simulink model "parallel"  (R2015b)
settings: Solver=FixedStepDiscrete  SolverMode=SingleTasking  StartTime=0.0  StopTime=600e-6  RelTol=1e-3
values from neighbouring files (symbols this model uses):
  b = ['00';'02';'04';'06';'08';'0a';'0c';'0e';'10';'12';'14';'16';'18';'1a';'1c';'1e';'20';'22';'24';'26';'28';'2a';'2c';'2e';'30';'32';'34';'36';'38';'3a';'3c';'3e';'40';'42';'44';'46';'48';'4a';'4c';'4e';'50';'52';'54';'56';'58';'5a';'5c';'5e';'60';'62';'64';'66';'68';'6a';'6c';'6e';'70';'72';'74';'76';'78';'7a';'7c';'7e';'80';'82';'84';'86';'88';'8a';'8c';'8e';'90';'92';'94';'96';'98';'9a';'9c';'9e' ...(+881 chars)    [parallelpipe_tb.m]
  input_sample_rate = 1.0E06    (= 1000000)    [parallelpipe_tb.m]
undefined symbols (not defined in the file or in its folder): a
libraries: shlslibv1 x6037
(part 40 of 40)

== system parallel/AES1 1/Round8/Subsystem8/Subsystem1/Mixcolumn2 ==
  In1 : Inport
  In2 : Inport  Port=2
  In3 : Inport  Port=3
  In4 : Inport  Port=4
  Binary Logic : shlslibv1/Math Functions/Binary Logic  syn_binlog_exp=a^b  synBlockType=primitive  synLatency=0  synBlockId=13
  Binary Logic1 : shlslibv1/Math Functions/Binary Logic  syn_binlog_exp=a^b  synBlockType=primitive  synLatency=0  synBlockId=13
  Binary Logic2 : shlslibv1/Math Functions/Binary Logic  syn_binlog_exp=a^b  synBlockType=primitive  synLatency=0  synBlockId=13
  Display5 : Display
      settings: Format=hex (Stored Integer)
  Port Out : shlslibv1/Ports & Subsystems/Port Out  syn_capture=on  syn_register=on  synBlockType=port  synLatency=1  synBlockId=1
  multiplier2 : shlslibv1/Memories/ROM  syn_rom_vec=multiplier2  syn_rom_auto_wl=on  syn_out_wl=8  syn_out_fl=0  syn_out_dt=unsigned  syn_out_sat=on  syn_out_rnd=on  syn_en_port=off  synBlockType=primitive  synLatency=1  synBlockId=62  syn_dual_port=off
  multiplier3 : shlslibv1/Memories/ROM  syn_rom_vec=multiplier3  syn_rom_auto_wl=on  syn_out_wl=8  syn_out_fl=0  syn_out_dt=unsigned  syn_out_sat=on  syn_out_rnd=on  syn_en_port=off  synBlockType=primitive  synLatency=1  synBlockId=62  syn_dual_port=off
  Out1 : Outport
  wires:
  In1/1 -> Binary Logic/1
  Binary Logic2/1 -> Port Out/1, Out1/1
  In4/1 -> multiplier3/1
  In3/1 -> multiplier2/1
  In2/1 -> Binary Logic/2
  multiplier2/1 -> Binary Logic1/1
  multiplier3/1 -> Binary Logic1/2
  Binary Logic/1 -> Binary Logic2/1
  Binary Logic1/1 -> Binary Logic2/2
  Port Out/1 -> Display5/1

== system parallel/AES1 1/Round8/Subsystem8/Subsystem1/Mixcolumn3 ==
  In1 : Inport
  In2 : Inport  Port=2
  In3 : Inport  Port=3
  In4 : Inport  Port=4
  Binary Logic : shlslibv1/Math Functions/Binary Logic  syn_binlog_exp=a^b  synBlockType=primitive  synLatency=0  synBlockId=13
  Binary Logic1 : shlslibv1/Math Functions/Binary Logic  syn_binlog_exp=a^b  synBlockType=primitive  synLatency=0  synBlockId=13
  Binary Logic2 : shlslibv1/Math Functions/Binary Logic  syn_binlog_exp=a^b  synBlockType=primitive  synLatency=0  synBlockId=13
  Display5 : Display
      settings: Format=hex (Stored Integer)
  Port Out : shlslibv1/Ports & Subsystems/Port Out  syn_capture=on  syn_register=on  synBlockType=port  synLatency=1  synBlockId=1
  multiplier1 : shlslibv1/Memories/ROM  syn_rom_vec=multiplier2  syn_rom_auto_wl=on  syn_out_wl=8  syn_out_fl=0  syn_out_dt=unsigned  syn_out_sat=on  syn_out_rnd=on  syn_en_port=off  synBlockType=primitive  synLatency=1  synBlockId=62  syn_dual_port=off
  multiplier4 : shlslibv1/Memories/ROM  syn_rom_vec=multiplier3  syn_rom_auto_wl=on  syn_out_wl=8  syn_out_fl=0  syn_out_dt=unsigned  syn_out_sat=on  syn_out_rnd=on  syn_en_port=off  synBlockType=primitive  synLatency=1  synBlockId=62  syn_dual_port=off
  Out1 : Outport
  wires:
  In2/1 -> Binary Logic/2
  multiplier1/1 -> Binary Logic1/2
  multiplier4/1 -> Binary Logic/1
  In3/1 -> Binary Logic1/1
  In1/1 -> multiplier4/1
  Binary Logic2/1 -> Port Out/1, Out1/1
  In4/1 -> multiplier1/1
  Port Out/1 -> Display5/1
  Binary Logic/1 -> Binary Logic2/1
  Binary Logic1/1 -> Binary Logic2/2

== system parallel/AES1 1/Round8/Subsystem8/Subsystem2/Mixcolumn ==
  In1 : Inport
  In2 : Inport  Port=2
  In3 : Inport  Port=3
  In4 : Inport  Port=4
  Binary Logic : shlslibv1/Math Functions/Binary Logic  syn_binlog_exp=a^b  synBlockType=primitive  synLatency=0  synBlockId=13
  Binary Logic1 : shlslibv1/Math Functions/Binary Logic  syn_binlog_exp=a^b  synBlockType=primitive  synLatency=0  synBlockId=13
  Binary Logic2 : shlslibv1/Math Functions/Binary Logic  syn_binlog_exp=a^b  synBlockType=primitive  synLatency=0  synBlockId=13
  Display5 : Display
      settings: Format=hex (Stored Integer)
  Port Out : shlslibv1/Ports & Subsystems/Port Out  syn_capture=on  syn_register=on  synBlockType=port  synLatency=1  synBlockId=1
  multiplier2 : shlslibv1/Memories/ROM  syn_rom_vec=multiplier2  syn_rom_auto_wl=on  syn_out_wl=8  syn_out_fl=0  syn_out_dt=unsigned  syn_out_sat=on  syn_out_rnd=on  syn_en_port=off  synBlockType=primitive  synLatency=1  synBlockId=62  syn_dual_port=off
  multiplier3 : shlslibv1/Memories/ROM  syn_rom_vec=multiplier3  syn_rom_auto_wl=on  syn_out_wl=8  syn_out_fl=0  syn_out_dt=unsigned  syn_out_sat=on  syn_out_rnd=on  syn_en_port=off  synBlockType=primitive  synLatency=1  synBlockId=62  syn_dual_port=off
  Out1 : Outport
  wires:
  multiplier3/1 -> Binary Logic/2
  In2/1 -> multiplier3/1
  In4/1 -> Binary Logic1/2
  multiplier2/1 -> Binary Logic/1
  In3/1 -> Binary Logic1/1
  Binary Logic2/1 -> Port Out/1, Out1/1
  In1/1 -> multiplier2/1
  Port Out/1 -> Display5/1
  Binary Logic/1 -> Binary Logic2/1
  Binary Logic1/1 -> Binary Logic2/2

== system parallel/AES1 1/Round8/Subsystem8/Subsystem2/Mixcolumn1 ==
  In1 : Inport
  In2 : Inport  Port=2
  In3 : Inport  Port=3
  In4 : Inport  Port=4
  Binary Logic : shlslibv1/Math Functions/Binary Logic  syn_binlog_exp=a^b  synBlockType=primitive  synLatency=0  synBlockId=13
  Binary Logic1 : shlslibv1/Math Functions/Binary Logic  syn_binlog_exp=a^b  synBlockType=primitive  synLatency=0  synBlockId=13
  Binary Logic2 : shlslibv1/Math Functions/Binary Logic  syn_binlog_exp=a^b  synBlockType=primitive  synLatency=0  synBlockId=13
  Display5 : Display
      settings: Format=hex (Stored Integer)
  Port Out : shlslibv1/Ports & Subsystems/Port Out  syn_capture=on  syn_register=on  synBlockType=port  synLatency=1  synBlockId=1
  multiplier2 : shlslibv1/Memories/ROM  syn_rom_vec=multiplier2  syn_rom_auto_wl=on  syn_out_wl=8  syn_out_fl=0  syn_out_dt=unsigned  syn_out_sat=on  syn_out_rnd=on  syn_en_port=off  synBlockType=primitive  synLatency=1  synBlockId=62  syn_dual_port=off
  multiplier4 : shlslibv1/Memories/ROM  syn_rom_vec=multiplier3  syn_rom_auto_wl=on  syn_out_wl=8  syn_out_fl=0  syn_out_dt=unsigned  syn_out_sat=on  syn_out_rnd=on  syn_en_port=off  synBlockType=primitive  synLatency=1  synBlockId=62  syn_dual_port=off
  Out1 : Outport
  wires:
  multiplier2/1 -> Binary Logic/2
  In2/1 -> multiplier2/1
  In4/1 -> Binary Logic1/2
  In1/1 -> Binary Logic/1
  multiplier4/1 -> Binary Logic1/1
  Binary Logic2/1 -> Port Out/1, Out1/1
  In3/1 -> multiplier4/1
  Port Out/1 -> Display5/1
  Binary Logic/1 -> Binary Logic2/1
  Binary Logic1/1 -> Binary Logic2/2

== system parallel/AES1 1/Round8/Subsystem8/Subsystem2/Mixcolumn2 ==
  In1 : Inport
  In2 : Inport  Port=2
  In3 : Inport  Port=3
  In4 : Inport  Port=4
  Binary Logic : shlslibv1/Math Functions/Binary Logic  syn_binlog_exp=a^b  synBlockType=primitive  synLatency=0  synBlockId=13
  Binary Logic1 : shlslibv1/Math Functions/Binary Logic  syn_binlog_exp=a^b  synBlockType=primitive  synLatency=0  synBlockId=13
  Binary Logic2 : shlslibv1/Math Functions/Binary Logic  syn_binlog_exp=a^b  synBlockType=primitive  synLatency=0  synBlockId=13
  Display5 : Display
      settings: Format=hex (Stored Integer)
  Port Out : shlslibv1/Ports & Subsystems/Port Out  syn_capture=on  syn_register=on  synBlockType=port  synLatency=1  synBlockId=1
  multiplier2 : shlslibv1/Memories/ROM  syn_rom_vec=multiplier2  syn_rom_auto_wl=on  syn_out_wl=8  syn_out_fl=0  syn_out_dt=unsigned  syn_out_sat=on  syn_out_rnd=on  syn_en_port=off  synBlockType=primitive  synLatency=1  synBlockId=62  syn_dual_port=off
  multiplier3 : shlslibv1/Memories/ROM  syn_rom_vec=multiplier3  syn_rom_auto_wl=on  syn_out_wl=8  syn_out_fl=0  syn_out_dt=unsigned  syn_out_sat=on  syn_out_rnd=on  syn_en_port=off  synBlockType=primitive  synLatency=1  synBlockId=62  syn_dual_port=off
  Out1 : Outport
  wires:
  In1/1 -> Binary Logic/1
  Binary Logic2/1 -> Port Out/1, Out1/1
  In4/1 -> multiplier3/1
  In3/1 -> multiplier2/1
  In2/1 -> Binary Logic/2
  multiplier2/1 -> Binary Logic1/1
  multiplier3/1 -> Binary Logic1/2
  Binary Logic/1 -> Binary Logic2/1
  Binary Logic1/1 -> Binary Logic2/2
  Port Out/1 -> Display5/1

== system parallel/AES1 1/Round8/Subsystem8/Subsystem2/Mixcolumn3 ==
  In1 : Inport
  In2 : Inport  Port=2
  In3 : Inport  Port=3
  In4 : Inport  Port=4
  Binary Logic : shlslibv1/Math Functions/Binary Logic  syn_binlog_exp=a^b  synBlockType=primitive  synLatency=0  synBlockId=13
  Binary Logic1 : shlslibv1/Math Functions/Binary Logic  syn_binlog_exp=a^b  synBlockType=primitive  synLatency=0  synBlockId=13
  Binary Logic2 : shlslibv1/Math Functions/Binary Logic  syn_binlog_exp=a^b  synBlockType=primitive  synLatency=0  synBlockId=13
  Display5 : Display
      settings: Format=hex (Stored Integer)
  Port Out : shlslibv1/Ports & Subsystems/Port Out  syn_capture=on  syn_register=on  synBlockType=port  synLatency=1  synBlockId=1
  multiplier1 : shlslibv1/Memories/ROM  syn_rom_vec=multiplier2  syn_rom_auto_wl=on  syn_out_wl=8  syn_out_fl=0  syn_out_dt=unsigned  syn_out_sat=on  syn_out_rnd=on  syn_en_port=off  synBlockType=primitive  synLatency=1  synBlockId=62  syn_dual_port=off
  multiplier4 : shlslibv1/Memories/ROM  syn_rom_vec=multiplier3  syn_rom_auto_wl=on  syn_out_wl=8  syn_out_fl=0  syn_out_dt=unsigned  syn_out_sat=on  syn_out_rnd=on  syn_en_port=off  synBlockType=primitive  synLatency=1  synBlockId=62  syn_dual_port=off
  Out1 : Outport
  wires:
  In2/1 -> Binary Logic/2
  multiplier1/1 -> Binary Logic1/2
  multiplier4/1 -> Binary Logic/1
  In3/1 -> Binary Logic1/1
  In1/1 -> multiplier4/1
  Binary Logic2/1 -> Port Out/1, Out1/1
  In4/1 -> multiplier1/1
  Port Out/1 -> Display5/1
  Binary Logic/1 -> Binary Logic2/1
  Binary Logic1/1 -> Binary Logic2/2

== system parallel/AES1 1/Round8/Subsystem8/Subsystem3/Mixcolumn ==
  In1 : Inport
  In2 : Inport  Port=2
  In3 : Inport  Port=3
  In4 : Inport  Port=4
  Binary Logic : shlslibv1/Math Functions/Binary Logic  syn_binlog_exp=a^b  synBlockType=primitive  synLatency=0  synBlockId=13
  Binary Logic1 : shlslibv1/Math Functions/Binary Logic  syn_binlog_exp=a^b  synBlockType=primitive  synLatency=0  synBlockId=13
  Binary Logic2 : shlslibv1/Math Functions/Binary Logic  syn_binlog_exp=a^b  synBlockType=primitive  synLatency=0  synBlockId=13
  Display5 : Display
      settings: Format=hex (Stored Integer)
  Port Out : shlslibv1/Ports & Subsystems/Port Out  syn_capture=on  syn_register=on  synBlockType=port  synLatency=1  synBlockId=1
  multiplier2 : shlslibv1/Memories/ROM  syn_rom_vec=multiplier2  syn_rom_auto_wl=on  syn_out_wl=8  syn_out_fl=0  syn_out_dt=unsigned  syn_out_sat=on  syn_out_rnd=on  syn_en_port=off  synBlockType=primitive  synLatency=1  synBlockId=62  syn_dual_port=off
  multiplier3 : shlslibv1/Memories/ROM  syn_rom_vec=multiplier3  syn_rom_auto_wl=on  syn_out_wl=8  syn_out_fl=0  syn_out_dt=unsigned  syn_out_sat=on  syn_out_rnd=on  syn_en_port=off  synBlockType=primitive  synLatency=1  synBlockId=62  syn_dual_port=off
  Out1 : Outport
  wires:
  multiplier3/1 -> Binary Logic/2
  In2/1 -> multiplier3/1
  In4/1 -> Binary Logic1/2
  multiplier2/1 -> Binary Logic/1
  In3/1 -> Binary Logic1/1
  Binary Logic2/1 -> Port Out/1, Out1/1
  In1/1 -> multiplier2/1
  Port Out/1 -> Display5/1
  Binary Logic/1 -> Binary Logic2/1
  Binary Logic1/1 -> Binary Logic2/2

== system parallel/AES1 1/Round8/Subsystem8/Subsystem3/Mixcolumn1 ==
  In1 : Inport
  In2 : Inport  Port=2
  In3 : Inport  Port=3
  In4 : Inport  Port=4
  Binary Logic : shlslibv1/Math Functions/Binary Logic  syn_binlog_exp=a^b  synBlockType=primitive  synLatency=0  synBlockId=13
  Binary Logic1 : shlslibv1/Math Functions/Binary Logic  syn_binlog_exp=a^b  synBlockType=primitive  synLatency=0  synBlockId=13
  Binary Logic2 : shlslibv1/Math Functions/Binary Logic  syn_binlog_exp=a^b  synBlockType=primitive  synLatency=0  synBlockId=13
  Display5 : Display
      settings: Format=hex (Stored Integer)
  Port Out : shlslibv1/Ports & Subsystems/Port Out  syn_capture=on  syn_register=on  synBlockType=port  synLatency=1  synBlockId=1
  multiplier2 : shlslibv1/Memories/ROM  syn_rom_vec=multiplier2  syn_rom_auto_wl=on  syn_out_wl=8  syn_out_fl=0  syn_out_dt=unsigned  syn_out_sat=on  syn_out_rnd=on  syn_en_port=off  synBlockType=primitive  synLatency=1  synBlockId=62  syn_dual_port=off
  multiplier4 : shlslibv1/Memories/ROM  syn_rom_vec=multiplier3  syn_rom_auto_wl=on  syn_out_wl=8  syn_out_fl=0  syn_out_dt=unsigned  syn_out_sat=on  syn_out_rnd=on  syn_en_port=off  synBlockType=primitive  synLatency=1  synBlockId=62  syn_dual_port=off
  Out1 : Outport
  wires:
  multiplier2/1 -> Binary Logic/2
  In2/1 -> multiplier2/1
  In4/1 -> Binary Logic1/2
  In1/1 -> Binary Logic/1
  multiplier4/1 -> Binary Logic1/1
  Binary Logic2/1 -> Port Out/1, Out1/1
  In3/1 -> multiplier4/1
  Port Out/1 -> Display5/1
  Binary Logic/1 -> Binary Logic2/1
  Binary Logic1/1 -> Binary Logic2/2

== system parallel/AES1 1/Round8/Subsystem8/Subsystem3/Mixcolumn2 ==
  In1 : Inport
  In2 : Inport  Port=2
  In3 : Inport  Port=3
  In4 : Inport  Port=4
  Binary Logic : shlslibv1/Math Functions/Binary Logic  syn_binlog_exp=a^b  synBlockType=primitive  synLatency=0  synBlockId=13
  Binary Logic1 : shlslibv1/Math Functions/Binary Logic  syn_binlog_exp=a^b  synBlockType=primitive  synLatency=0  synBlockId=13
  Binary Logic2 : shlslibv1/Math Functions/Binary Logic  syn_binlog_exp=a^b  synBlockType=primitive  synLatency=0  synBlockId=13
  Display5 : Display
      settings: Format=hex (Stored Integer)
  Port Out : shlslibv1/Ports & Subsystems/Port Out  syn_capture=on  syn_register=on  synBlockType=port  synLatency=1  synBlockId=1
  multiplier2 : shlslibv1/Memories/ROM  syn_rom_vec=multiplier2  syn_rom_auto_wl=on  syn_out_wl=8  syn_out_fl=0  syn_out_dt=unsigned  syn_out_sat=on  syn_out_rnd=on  syn_en_port=off  synBlockType=primitive  synLatency=1  synBlockId=62  syn_dual_port=off
  multiplier3 : shlslibv1/Memories/ROM  syn_rom_vec=multiplier3  syn_rom_auto_wl=on  syn_out_wl=8  syn_out_fl=0  syn_out_dt=unsigned  syn_out_sat=on  syn_out_rnd=on  syn_en_port=off  synBlockType=primitive  synLatency=1  synBlockId=62  syn_dual_port=off
  Out1 : Outport
  wires:
  In1/1 -> Binary Logic/1
  Binary Logic2/1 -> Port Out/1, Out1/1
  In4/1 -> multiplier3/1
  In3/1 -> multiplier2/1
  In2/1 -> Binary Logic/2
  multiplier2/1 -> Binary Logic1/1
  multiplier3/1 -> Binary Logic1/2
  Binary Logic/1 -> Binary Logic2/1
  Binary Logic1/1 -> Binary Logic2/2
  Port Out/1 -> Display5/1

== system parallel/AES1 1/Round8/Subsystem8/Subsystem3/Mixcolumn3 ==
  In1 : Inport
  In2 : Inport  Port=2
  In3 : Inport  Port=3
  In4 : Inport  Port=4
  Binary Logic : shlslibv1/Math Functions/Binary Logic  syn_binlog_exp=a^b  synBlockType=primitive  synLatency=0  synBlockId=13
  Binary Logic1 : shlslibv1/Math Functions/Binary Logic  syn_binlog_exp=a^b  synBlockType=primitive  synLatency=0  synBlockId=13
  Binary Logic2 : shlslibv1/Math Functions/Binary Logic  syn_binlog_exp=a^b  synBlockType=primitive  synLatency=0  synBlockId=13
  Display5 : Display
      settings: Format=hex (Stored Integer)
  Port Out : shlslibv1/Ports & Subsystems/Port Out  syn_capture=on  syn_register=on  synBlockType=port  synLatency=1  synBlockId=1
  multiplier1 : shlslibv1/Memories/ROM  syn_rom_vec=multiplier2  syn_rom_auto_wl=on  syn_out_wl=8  syn_out_fl=0  syn_out_dt=unsigned  syn_out_sat=on  syn_out_rnd=on  syn_en_port=off  synBlockType=primitive  synLatency=1  synBlockId=62  syn_dual_port=off
  multiplier4 : shlslibv1/Memories/ROM  syn_rom_vec=multiplier3  syn_rom_auto_wl=on  syn_out_wl=8  syn_out_fl=0  syn_out_dt=unsigned  syn_out_sat=on  syn_out_rnd=on  syn_en_port=off  synBlockType=primitive  synLatency=1  synBlockId=62  syn_dual_port=off
  Out1 : Outport
  wires:
  In2/1 -> Binary Logic/2
  multiplier1/1 -> Binary Logic1/2
  multiplier4/1 -> Binary Logic/1
  In3/1 -> Binary Logic1/1
  In1/1 -> multiplier4/1
  Binary Logic2/1 -> Port Out/1, Out1/1
  In4/1 -> multiplier1/1
  Port Out/1 -> Display5/1
  Binary Logic/1 -> Binary Logic2/1
  Binary Logic1/1 -> Binary Logic2/2

== system parallel/AES1 1/Round9/Key1/Keygen1/Subsystem4 ==
  In1 : Inport
  In2 : Inport  Port=2
  In3 : Inport  Port=3
  In4 : Inport  Port=4
  ROM{1..4} (4 alike) : shlslibv1/Memories/ROM  syn_rom_vec=sbox  syn_rom_auto_wl=on  syn_out_wl=8  syn_out_fl=0  syn_out_dt=unsigned  syn_out_sat=on  syn_out_rnd=on  syn_en_port=off  synBlockType=primitive  synLatency=1  synBlockId=62  syn_dual_port=off
  Out1 : Outport
  Out2 : Outport  Port=2
  Out3 : Outport  Port=3
  Out4 : Outport  Port=4
  wires:
  In1/1 -> ROM4/1
  In4/1 -> ROM3/1
  In3/1 -> ROM2/1
  ROM4/1 -> Out1/1
  ROM1/1 -> Out2/1
  ROM2/1 -> Out3/1
  ROM3/1 -> Out4/1
  In2/1 -> ROM1/1

== system parallel/AES1 1/Round9/Subsystem8/Subsystem/Mixcolumn ==
  In1 : Inport
  In2 : Inport  Port=2
  In3 : Inport  Port=3
  In4 : Inport  Port=4
  Binary Logic : shlslibv1/Math Functions/Binary Logic  syn_binlog_exp=a^b  synBlockType=primitive  synLatency=0  synBlockId=13
  Binary Logic1 : shlslibv1/Math Functions/Binary Logic  syn_binlog_exp=a^b  synBlockType=primitive  synLatency=0  synBlockId=13
  Binary Logic2 : shlslibv1/Math Functions/Binary Logic  syn_binlog_exp=a^b  synBlockType=primitive  synLatency=0  synBlockId=13
  Display5 : Display
      settings: Format=hex (Stored Integer)
  Port Out : shlslibv1/Ports & Subsystems/Port Out  syn_capture=on  syn_register=on  synBlockType=port  synLatency=1  synBlockId=1
  multiplier2 : shlslibv1/Memories/ROM  syn_rom_vec=multiplier2  syn_rom_auto_wl=on  syn_out_wl=8  syn_out_fl=0  syn_out_dt=unsigned  syn_out_sat=on  syn_out_rnd=on  syn_en_port=off  synBlockType=primitive  synLatency=1  synBlockId=62  syn_dual_port=off
  multiplier3 : shlslibv1/Memories/ROM  syn_rom_vec=multiplier3  syn_rom_auto_wl=on  syn_out_wl=8  syn_out_fl=0  syn_out_dt=unsigned  syn_out_sat=on  syn_out_rnd=on  syn_en_port=off  synBlockType=primitive  synLatency=1  synBlockId=62  syn_dual_port=off
  Out1 : Outport
  wires:
  multiplier3/1 -> Binary Logic/2
  In2/1 -> multiplier3/1
  In4/1 -> Binary Logic1/2
  multiplier2/1 -> Binary Logic/1
  In3/1 -> Binary Logic1/1
  Binary Logic2/1 -> Port Out/1, Out1/1
  In1/1 -> multiplier2/1
  Port Out/1 -> Display5/1
  Binary Logic/1 -> Binary Logic2/1
  Binary Logic1/1 -> Binary Logic2/2

== system parallel/AES1 1/Round9/Subsystem8/Subsystem/Mixcolumn1 ==
  In1 : Inport
  In2 : Inport  Port=2
  In3 : Inport  Port=3
  In4 : Inport  Port=4
  Binary Logic : shlslibv1/Math Functions/Binary Logic  syn_binlog_exp=a^b  synBlockType=primitive  synLatency=0  synBlockId=13
  Binary Logic1 : shlslibv1/Math Functions/Binary Logic  syn_binlog_exp=a^b  synBlockType=primitive  synLatency=0  synBlockId=13
  Binary Logic2 : shlslibv1/Math Functions/Binary Logic  syn_binlog_exp=a^b  synBlockType=primitive  synLatency=0  synBlockId=13
  Display5 : Display
      settings: Format=hex (Stored Integer)
  Port Out : shlslibv1/Ports & Subsystems/Port Out  syn_capture=on  syn_register=on  synBlockType=port  synLatency=1  synBlockId=1
  multiplier2 : shlslibv1/Memories/ROM  syn_rom_vec=multiplier2  syn_rom_auto_wl=on  syn_out_wl=8  syn_out_fl=0  syn_out_dt=unsigned  syn_out_sat=on  syn_out_rnd=on  syn_en_port=off  synBlockType=primitive  synLatency=1  synBlockId=62  syn_dual_port=off
  multiplier4 : shlslibv1/Memories/ROM  syn_rom_vec=multiplier3  syn_rom_auto_wl=on  syn_out_wl=8  syn_out_fl=0  syn_out_dt=unsigned  syn_out_sat=on  syn_out_rnd=on  syn_en_port=off  synBlockType=primitive  synLatency=1  synBlockId=62  syn_dual_port=off
  Out1 : Outport
  wires:
  multiplier2/1 -> Binary Logic/2
  In2/1 -> multiplier2/1
  In4/1 -> Binary Logic1/2
  In1/1 -> Binary Logic/1
  multiplier4/1 -> Binary Logic1/1
  Binary Logic2/1 -> Port Out/1, Out1/1
  In3/1 -> multiplier4/1
  Port Out/1 -> Display5/1
  Binary Logic/1 -> Binary Logic2/1
  Binary Logic1/1 -> Binary Logic2/2

== system parallel/AES1 1/Round9/Subsystem8/Subsystem/Mixcolumn2 ==
  In1 : Inport
  In2 : Inport  Port=2
  In3 : Inport  Port=3
  In4 : Inport  Port=4
  Binary Logic : shlslibv1/Math Functions/Binary Logic  syn_binlog_exp=a^b  synBlockType=primitive  synLatency=0  synBlockId=13
  Binary Logic1 : shlslibv1/Math Functions/Binary Logic  syn_binlog_exp=a^b  synBlockType=primitive  synLatency=0  synBlockId=13
  Binary Logic2 : shlslibv1/Math Functions/Binary Logic  syn_binlog_exp=a^b  synBlockType=primitive  synLatency=0  synBlockId=13
  Display5 : Display
      settings: Format=hex (Stored Integer)
  Port Out : shlslibv1/Ports & Subsystems/Port Out  syn_capture=on  syn_register=on  synBlockType=port  synLatency=1  synBlockId=1
  multiplier2 : shlslibv1/Memories/ROM  syn_rom_vec=multiplier2  syn_rom_auto_wl=on  syn_out_wl=8  syn_out_fl=0  syn_out_dt=unsigned  syn_out_sat=on  syn_out_rnd=on  syn_en_port=off  synBlockType=primitive  synLatency=1  synBlockId=62  syn_dual_port=off
  multiplier3 : shlslibv1/Memories/ROM  syn_rom_vec=multiplier3  syn_rom_auto_wl=on  syn_out_wl=8  syn_out_fl=0  syn_out_dt=unsigned  syn_out_sat=on  syn_out_rnd=on  syn_en_port=off  synBlockType=primitive  synLatency=1  synBlockId=62  syn_dual_port=off
  Out1 : Outport
  wires:
  In1/1 -> Binary Logic/1
  Binary Logic2/1 -> Port Out/1, Out1/1
  In4/1 -> multiplier3/1
  In3/1 -> multiplier2/1
  In2/1 -> Binary Logic/2
  multiplier2/1 -> Binary Logic1/1
  multiplier3/1 -> Binary Logic1/2
  Binary Logic/1 -> Binary Logic2/1
  Binary Logic1/1 -> Binary Logic2/2
  Port Out/1 -> Display5/1

== system parallel/AES1 1/Round9/Subsystem8/Subsystem/Mixcolumn3 ==
  In1 : Inport
  In2 : Inport  Port=2
  In3 : Inport  Port=3
  In4 : Inport  Port=4
  Binary Logic : shlslibv1/Math Functions/Binary Logic  syn_binlog_exp=a^b  synBlockType=primitive  synLatency=0  synBlockId=13
  Binary Logic1 : shlslibv1/Math Functions/Binary Logic  syn_binlog_exp=a^b  synBlockType=primitive  synLatency=0  synBlockId=13
  Binary Logic2 : shlslibv1/Math Functions/Binary Logic  syn_binlog_exp=a^b  synBlockType=primitive  synLatency=0  synBlockId=13
  Display5 : Display
      settings: Format=hex (Stored Integer)
  Port Out : shlslibv1/Ports & Subsystems/Port Out  syn_capture=on  syn_register=on  synBlockType=port  synLatency=1  synBlockId=1
  multiplier1 : shlslibv1/Memories/ROM  syn_rom_vec=multiplier2  syn_rom_auto_wl=on  syn_out_wl=8  syn_out_fl=0  syn_out_dt=unsigned  syn_out_sat=on  syn_out_rnd=on  syn_en_port=off  synBlockType=primitive  synLatency=1  synBlockId=62  syn_dual_port=off
  multiplier4 : shlslibv1/Memories/ROM  syn_rom_vec=multiplier3  syn_rom_auto_wl=on  syn_out_wl=8  syn_out_fl=0  syn_out_dt=unsigned  syn_out_sat=on  syn_out_rnd=on  syn_en_port=off  synBlockType=primitive  synLatency=1  synBlockId=62  syn_dual_port=off
  Out1 : Outport
  wires:
  In2/1 -> Binary Logic/2
  multiplier1/1 -> Binary Logic1/2
  multiplier4/1 -> Binary Logic/1
  In3/1 -> Binary Logic1/1
  In1/1 -> multiplier4/1
  Binary Logic2/1 -> Port Out/1, Out1/1
  In4/1 -> multiplier1/1
  Port Out/1 -> Display5/1
  Binary Logic/1 -> Binary Logic2/1
  Binary Logic1/1 -> Binary Logic2/2

== system parallel/AES1 1/Round9/Subsystem8/Subsystem1/Mixcolumn ==
  In1 : Inport
  In2 : Inport  Port=2
  In3 : Inport  Port=3
  In4 : Inport  Port=4
  Binary Logic : shlslibv1/Math Functions/Binary Logic  syn_binlog_exp=a^b  synBlockType=primitive  synLatency=0  synBlockId=13
  Binary Logic1 : shlslibv1/Math Functions/Binary Logic  syn_binlog_exp=a^b  synBlockType=primitive  synLatency=0  synBlockId=13
  Binary Logic2 : shlslibv1/Math Functions/Binary Logic  syn_binlog_exp=a^b  synBlockType=primitive  synLatency=0  synBlockId=13
  Display5 : Display
      settings: Format=hex (Stored Integer)
  Port Out : shlslibv1/Ports & Subsystems/Port Out  syn_capture=on  syn_register=on  synBlockType=port  synLatency=1  synBlockId=1
  multiplier2 : shlslibv1/Memories/ROM  syn_rom_vec=multiplier2  syn_rom_auto_wl=on  syn_out_wl=8  syn_out_fl=0  syn_out_dt=unsigned  syn_out_sat=on  syn_out_rnd=on  syn_en_port=off  synBlockType=primitive  synLatency=1  synBlockId=62  syn_dual_port=off
  multiplier3 : shlslibv1/Memories/ROM  syn_rom_vec=multiplier3  syn_rom_auto_wl=on  syn_out_wl=8  syn_out_fl=0  syn_out_dt=unsigned  syn_out_sat=on  syn_out_rnd=on  syn_en_port=off  synBlockType=primitive  synLatency=1  synBlockId=62  syn_dual_port=off
  Out1 : Outport
  wires:
  multiplier3/1 -> Binary Logic/2
  In2/1 -> multiplier3/1
  In4/1 -> Binary Logic1/2
  multiplier2/1 -> Binary Logic/1
  In3/1 -> Binary Logic1/1
  Binary Logic2/1 -> Port Out/1, Out1/1
  In1/1 -> multiplier2/1
  Port Out/1 -> Display5/1
  Binary Logic/1 -> Binary Logic2/1
  Binary Logic1/1 -> Binary Logic2/2

== system parallel/AES1 1/Round9/Subsystem8/Subsystem1/Mixcolumn1 ==
  In1 : Inport
  In2 : Inport  Port=2
  In3 : Inport  Port=3
  In4 : Inport  Port=4
  Binary Logic : shlslibv1/Math Functions/Binary Logic  syn_binlog_exp=a^b  synBlockType=primitive  synLatency=0  synBlockId=13
  Binary Logic1 : shlslibv1/Math Functions/Binary Logic  syn_binlog_exp=a^b  synBlockType=primitive  synLatency=0  synBlockId=13
  Binary Logic2 : shlslibv1/Math Functions/Binary Logic  syn_binlog_exp=a^b  synBlockType=primitive  synLatency=0  synBlockId=13
  Display5 : Display
      settings: Format=hex (Stored Integer)
  Port Out : shlslibv1/Ports & Subsystems/Port Out  syn_capture=on  syn_register=on  synBlockType=port  synLatency=1  synBlockId=1
  multiplier2 : shlslibv1/Memories/ROM  syn_rom_vec=multiplier2  syn_rom_auto_wl=on  syn_out_wl=8  syn_out_fl=0  syn_out_dt=unsigned  syn_out_sat=on  syn_out_rnd=on  syn_en_port=off  synBlockType=primitive  synLatency=1  synBlockId=62  syn_dual_port=off
  multiplier4 : shlslibv1/Memories/ROM  syn_rom_vec=multiplier3  syn_rom_auto_wl=on  syn_out_wl=8  syn_out_fl=0  syn_out_dt=unsigned  syn_out_sat=on  syn_out_rnd=on  syn_en_port=off  synBlockType=primitive  synLatency=1  synBlockId=62  syn_dual_port=off
  Out1 : Outport
  wires:
  multiplier2/1 -> Binary Logic/2
  In2/1 -> multiplier2/1
  In4/1 -> Binary Logic1/2
  In1/1 -> Binary Logic/1
  multiplier4/1 -> Binary Logic1/1
  Binary Logic2/1 -> Port Out/1, Out1/1
  In3/1 -> multiplier4/1
  Port Out/1 -> Display5/1
  Binary Logic/1 -> Binary Logic2/1
  Binary Logic1/1 -> Binary Logic2/2

== system parallel/AES1 1/Round9/Subsystem8/Subsystem1/Mixcolumn2 ==
  In1 : Inport
  In2 : Inport  Port=2
  In3 : Inport  Port=3
  In4 : Inport  Port=4
  Binary Logic : shlslibv1/Math Functions/Binary Logic  syn_binlog_exp=a^b  synBlockType=primitive  synLatency=0  synBlockId=13
  Binary Logic1 : shlslibv1/Math Functions/Binary Logic  syn_binlog_exp=a^b  synBlockType=primitive  synLatency=0  synBlockId=13
  Binary Logic2 : shlslibv1/Math Functions/Binary Logic  syn_binlog_exp=a^b  synBlockType=primitive  synLatency=0  synBlockId=13
  Display5 : Display
      settings: Format=hex (Stored Integer)
  Port Out : shlslibv1/Ports & Subsystems/Port Out  syn_capture=on  syn_register=on  synBlockType=port  synLatency=1  synBlockId=1
  multiplier2 : shlslibv1/Memories/ROM  syn_rom_vec=multiplier2  syn_rom_auto_wl=on  syn_out_wl=8  syn_out_fl=0  syn_out_dt=unsigned  syn_out_sat=on  syn_out_rnd=on  syn_en_port=off  synBlockType=primitive  synLatency=1  synBlockId=62  syn_dual_port=off
  multiplier3 : shlslibv1/Memories/ROM  syn_rom_vec=multiplier3  syn_rom_auto_wl=on  syn_out_wl=8  syn_out_fl=0  syn_out_dt=unsigned  syn_out_sat=on  syn_out_rnd=on  syn_en_port=off  synBlockType=primitive  synLatency=1  synBlockId=62  syn_dual_port=off
  Out1 : Outport
  wires:
  In1/1 -> Binary Logic/1
  Binary Logic2/1 -> Port Out/1, Out1/1
  In4/1 -> multiplier3/1
  In3/1 -> multiplier2/1
  In2/1 -> Binary Logic/2
  multiplier2/1 -> Binary Logic1/1
  multiplier3/1 -> Binary Logic1/2
  Binary Logic/1 -> Binary Logic2/1
  Binary Logic1/1 -> Binary Logic2/2
  Port Out/1 -> Display5/1

== system parallel/AES1 1/Round9/Subsystem8/Subsystem1/Mixcolumn3 ==
  In1 : Inport
  In2 : Inport  Port=2
  In3 : Inport  Port=3
  In4 : Inport  Port=4
  Binary Logic : shlslibv1/Math Functions/Binary Logic  syn_binlog_exp=a^b  synBlockType=primitive  synLatency=0  synBlockId=13
  Binary Logic1 : shlslibv1/Math Functions/Binary Logic  syn_binlog_exp=a^b  synBlockType=primitive  synLatency=0  synBlockId=13
  Binary Logic2 : shlslibv1/Math Functions/Binary Logic  syn_binlog_exp=a^b  synBlockType=primitive  synLatency=0  synBlockId=13
  Display5 : Display
      settings: Format=hex (Stored Integer)
  Port Out : shlslibv1/Ports & Subsystems/Port Out  syn_capture=on  syn_register=on  synBlockType=port  synLatency=1  synBlockId=1
  multiplier1 : shlslibv1/Memories/ROM  syn_rom_vec=multiplier2  syn_rom_auto_wl=on  syn_out_wl=8  syn_out_fl=0  syn_out_dt=unsigned  syn_out_sat=on  syn_out_rnd=on  syn_en_port=off  synBlockType=primitive  synLatency=1  synBlockId=62  syn_dual_port=off
  multiplier4 : shlslibv1/Memories/ROM  syn_rom_vec=multiplier3  syn_rom_auto_wl=on  syn_out_wl=8  syn_out_fl=0  syn_out_dt=unsigned  syn_out_sat=on  syn_out_rnd=on  syn_en_port=off  synBlockType=primitive  synLatency=1  synBlockId=62  syn_dual_port=off
  Out1 : Outport
  wires:
  In2/1 -> Binary Logic/2
  multiplier1/1 -> Binary Logic1/2
  multiplier4/1 -> Binary Logic/1
  In3/1 -> Binary Logic1/1
  In1/1 -> multiplier4/1
  Binary Logic2/1 -> Port Out/1, Out1/1
  In4/1 -> multiplier1/1
  Port Out/1 -> Display5/1
  Binary Logic/1 -> Binary Logic2/1
  Binary Logic1/1 -> Binary Logic2/2

== system parallel/AES1 1/Round9/Subsystem8/Subsystem2/Mixcolumn ==
  In1 : Inport
  In2 : Inport  Port=2
  In3 : Inport  Port=3
  In4 : Inport  Port=4
  Binary Logic : shlslibv1/Math Functions/Binary Logic  syn_binlog_exp=a^b  synBlockType=primitive  synLatency=0  synBlockId=13
  Binary Logic1 : shlslibv1/Math Functions/Binary Logic  syn_binlog_exp=a^b  synBlockType=primitive  synLatency=0  synBlockId=13
  Binary Logic2 : shlslibv1/Math Functions/Binary Logic  syn_binlog_exp=a^b  synBlockType=primitive  synLatency=0  synBlockId=13
  Display5 : Display
      settings: Format=hex (Stored Integer)
  Port Out : shlslibv1/Ports & Subsystems/Port Out  syn_capture=on  syn_register=on  synBlockType=port  synLatency=1  synBlockId=1
  multiplier2 : shlslibv1/Memories/ROM  syn_rom_vec=multiplier2  syn_rom_auto_wl=on  syn_out_wl=8  syn_out_fl=0  syn_out_dt=unsigned  syn_out_sat=on  syn_out_rnd=on  syn_en_port=off  synBlockType=primitive  synLatency=1  synBlockId=62  syn_dual_port=off
  multiplier3 : shlslibv1/Memories/ROM  syn_rom_vec=multiplier3  syn_rom_auto_wl=on  syn_out_wl=8  syn_out_fl=0  syn_out_dt=unsigned  syn_out_sat=on  syn_out_rnd=on  syn_en_port=off  synBlockType=primitive  synLatency=1  synBlockId=62  syn_dual_port=off
  Out1 : Outport
  wires:
  multiplier3/1 -> Binary Logic/2
  In2/1 -> multiplier3/1
  In4/1 -> Binary Logic1/2
  multiplier2/1 -> Binary Logic/1
  In3/1 -> Binary Logic1/1
  Binary Logic2/1 -> Port Out/1, Out1/1
  In1/1 -> multiplier2/1
  Port Out/1 -> Display5/1
  Binary Logic/1 -> Binary Logic2/1
  Binary Logic1/1 -> Binary Logic2/2

== system parallel/AES1 1/Round9/Subsystem8/Subsystem2/Mixcolumn1 ==
  In1 : Inport
  In2 : Inport  Port=2
  In3 : Inport  Port=3
  In4 : Inport  Port=4
  Binary Logic : shlslibv1/Math Functions/Binary Logic  syn_binlog_exp=a^b  synBlockType=primitive  synLatency=0  synBlockId=13
  Binary Logic1 : shlslibv1/Math Functions/Binary Logic  syn_binlog_exp=a^b  synBlockType=primitive  synLatency=0  synBlockId=13
  Binary Logic2 : shlslibv1/Math Functions/Binary Logic  syn_binlog_exp=a^b  synBlockType=primitive  synLatency=0  synBlockId=13
  Display5 : Display
      settings: Format=hex (Stored Integer)
  Port Out : shlslibv1/Ports & Subsystems/Port Out  syn_capture=on  syn_register=on  synBlockType=port  synLatency=1  synBlockId=1
  multiplier2 : shlslibv1/Memories/ROM  syn_rom_vec=multiplier2  syn_rom_auto_wl=on  syn_out_wl=8  syn_out_fl=0  syn_out_dt=unsigned  syn_out_sat=on  syn_out_rnd=on  syn_en_port=off  synBlockType=primitive  synLatency=1  synBlockId=62  syn_dual_port=off
  multiplier4 : shlslibv1/Memories/ROM  syn_rom_vec=multiplier3  syn_rom_auto_wl=on  syn_out_wl=8  syn_out_fl=0  syn_out_dt=unsigned  syn_out_sat=on  syn_out_rnd=on  syn_en_port=off  synBlockType=primitive  synLatency=1  synBlockId=62  syn_dual_port=off
  Out1 : Outport
  wires:
  multiplier2/1 -> Binary Logic/2
  In2/1 -> multiplier2/1
  In4/1 -> Binary Logic1/2
  In1/1 -> Binary Logic/1
  multiplier4/1 -> Binary Logic1/1
  Binary Logic2/1 -> Port Out/1, Out1/1
  In3/1 -> multiplier4/1
  Port Out/1 -> Display5/1
  Binary Logic/1 -> Binary Logic2/1
  Binary Logic1/1 -> Binary Logic2/2

== system parallel/AES1 1/Round9/Subsystem8/Subsystem2/Mixcolumn2 ==
  In1 : Inport
  In2 : Inport  Port=2
  In3 : Inport  Port=3
  In4 : Inport  Port=4
  Binary Logic : shlslibv1/Math Functions/Binary Logic  syn_binlog_exp=a^b  synBlockType=primitive  synLatency=0  synBlockId=13
  Binary Logic1 : shlslibv1/Math Functions/Binary Logic  syn_binlog_exp=a^b  synBlockType=primitive  synLatency=0  synBlockId=13
  Binary Logic2 : shlslibv1/Math Functions/Binary Logic  syn_binlog_exp=a^b  synBlockType=primitive  synLatency=0  synBlockId=13
  Display5 : Display
      settings: Format=hex (Stored Integer)
  Port Out : shlslibv1/Ports & Subsystems/Port Out  syn_capture=on  syn_register=on  synBlockType=port  synLatency=1  synBlockId=1
  multiplier2 : shlslibv1/Memories/ROM  syn_rom_vec=multiplier2  syn_rom_auto_wl=on  syn_out_wl=8  syn_out_fl=0  syn_out_dt=unsigned  syn_out_sat=on  syn_out_rnd=on  syn_en_port=off  synBlockType=primitive  synLatency=1  synBlockId=62  syn_dual_port=off
  multiplier3 : shlslibv1/Memories/ROM  syn_rom_vec=multiplier3  syn_rom_auto_wl=on  syn_out_wl=8  syn_out_fl=0  syn_out_dt=unsigned  syn_out_sat=on  syn_out_rnd=on  syn_en_port=off  synBlockType=primitive  synLatency=1  synBlockId=62  syn_dual_port=off
  Out1 : Outport
  wires:
  In1/1 -> Binary Logic/1
  Binary Logic2/1 -> Port Out/1, Out1/1
  In4/1 -> multiplier3/1
  In3/1 -> multiplier2/1
  In2/1 -> Binary Logic/2
  multiplier2/1 -> Binary Logic1/1
  multiplier3/1 -> Binary Logic1/2
  Binary Logic/1 -> Binary Logic2/1
  Binary Logic1/1 -> Binary Logic2/2
  Port Out/1 -> Display5/1

== system parallel/AES1 1/Round9/Subsystem8/Subsystem2/Mixcolumn3 ==
  In1 : Inport
  In2 : Inport  Port=2
  In3 : Inport  Port=3
  In4 : Inport  Port=4
  Binary Logic : shlslibv1/Math Functions/Binary Logic  syn_binlog_exp=a^b  synBlockType=primitive  synLatency=0  synBlockId=13
  Binary Logic1 : shlslibv1/Math Functions/Binary Logic  syn_binlog_exp=a^b  synBlockType=primitive  synLatency=0  synBlockId=13
  Binary Logic2 : shlslibv1/Math Functions/Binary Logic  syn_binlog_exp=a^b  synBlockType=primitive  synLatency=0  synBlockId=13
  Display5 : Display
      settings: Format=hex (Stored Integer)
  Port Out : shlslibv1/Ports & Subsystems/Port Out  syn_capture=on  syn_register=on  synBlockType=port  synLatency=1  synBlockId=1
  multiplier1 : shlslibv1/Memories/ROM  syn_rom_vec=multiplier2  syn_rom_auto_wl=on  syn_out_wl=8  syn_out_fl=0  syn_out_dt=unsigned  syn_out_sat=on  syn_out_rnd=on  syn_en_port=off  synBlockType=primitive  synLatency=1  synBlockId=62  syn_dual_port=off
  multiplier4 : shlslibv1/Memories/ROM  syn_rom_vec=multiplier3  syn_rom_auto_wl=on  syn_out_wl=8  syn_out_fl=0  syn_out_dt=unsigned  syn_out_sat=on  syn_out_rnd=on  syn_en_port=off  synBlockType=primitive  synLatency=1  synBlockId=62  syn_dual_port=off
  Out1 : Outport
  wires:
  In2/1 -> Binary Logic/2
  multiplier1/1 -> Binary Logic1/2
  multiplier4/1 -> Binary Logic/1
  In3/1 -> Binary Logic1/1
  In1/1 -> multiplier4/1
  Binary Logic2/1 -> Port Out/1, Out1/1
  In4/1 -> multiplier1/1
  Port Out/1 -> Display5/1
  Binary Logic/1 -> Binary Logic2/1
  Binary Logic1/1 -> Binary Logic2/2

== system parallel/AES1 1/Round9/Subsystem8/Subsystem3/Mixcolumn ==
  In1 : Inport
  In2 : Inport  Port=2
  In3 : Inport  Port=3
  In4 : Inport  Port=4
  Binary Logic : shlslibv1/Math Functions/Binary Logic  syn_binlog_exp=a^b  synBlockType=primitive  synLatency=0  synBlockId=13
  Binary Logic1 : shlslibv1/Math Functions/Binary Logic  syn_binlog_exp=a^b  synBlockType=primitive  synLatency=0  synBlockId=13
  Binary Logic2 : shlslibv1/Math Functions/Binary Logic  syn_binlog_exp=a^b  synBlockType=primitive  synLatency=0  synBlockId=13
  Display5 : Display
      settings: Format=hex (Stored Integer)
  Port Out : shlslibv1/Ports & Subsystems/Port Out  syn_capture=on  syn_register=on  synBlockType=port  synLatency=1  synBlockId=1
  multiplier2 : shlslibv1/Memories/ROM  syn_rom_vec=multiplier2  syn_rom_auto_wl=on  syn_out_wl=8  syn_out_fl=0  syn_out_dt=unsigned  syn_out_sat=on  syn_out_rnd=on  syn_en_port=off  synBlockType=primitive  synLatency=1  synBlockId=62  syn_dual_port=off
  multiplier3 : shlslibv1/Memories/ROM  syn_rom_vec=multiplier3  syn_rom_auto_wl=on  syn_out_wl=8  syn_out_fl=0  syn_out_dt=unsigned  syn_out_sat=on  syn_out_rnd=on  syn_en_port=off  synBlockType=primitive  synLatency=1  synBlockId=62  syn_dual_port=off
  Out1 : Outport
  wires:
  multiplier3/1 -> Binary Logic/2
  In2/1 -> multiplier3/1
  In4/1 -> Binary Logic1/2
  multiplier2/1 -> Binary Logic/1
  In3/1 -> Binary Logic1/1
  Binary Logic2/1 -> Port Out/1, Out1/1
  In1/1 -> multiplier2/1
  Port Out/1 -> Display5/1
  Binary Logic/1 -> Binary Logic2/1
  Binary Logic1/1 -> Binary Logic2/2

== system parallel/AES1 1/Round9/Subsystem8/Subsystem3/Mixcolumn1 ==
  In1 : Inport
  In2 : Inport  Port=2
  In3 : Inport  Port=3
  In4 : Inport  Port=4
  Binary Logic : shlslibv1/Math Functions/Binary Logic  syn_binlog_exp=a^b  synBlockType=primitive  synLatency=0  synBlockId=13
  Binary Logic1 : shlslibv1/Math Functions/Binary Logic  syn_binlog_exp=a^b  synBlockType=primitive  synLatency=0  synBlockId=13
  Binary Logic2 : shlslibv1/Math Functions/Binary Logic  syn_binlog_exp=a^b  synBlockType=primitive  synLatency=0  synBlockId=13
  Display5 : Display
      settings: Format=hex (Stored Integer)
  Port Out : shlslibv1/Ports & Subsystems/Port Out  syn_capture=on  syn_register=on  synBlockType=port  synLatency=1  synBlockId=1
  multiplier2 : shlslibv1/Memories/ROM  syn_rom_vec=multiplier2  syn_rom_auto_wl=on  syn_out_wl=8  syn_out_fl=0  syn_out_dt=unsigned  syn_out_sat=on  syn_out_rnd=on  syn_en_port=off  synBlockType=primitive  synLatency=1  synBlockId=62  syn_dual_port=off
  multiplier4 : shlslibv1/Memories/ROM  syn_rom_vec=multiplier3  syn_rom_auto_wl=on  syn_out_wl=8  syn_out_fl=0  syn_out_dt=unsigned  syn_out_sat=on  syn_out_rnd=on  syn_en_port=off  synBlockType=primitive  synLatency=1  synBlockId=62  syn_dual_port=off
  Out1 : Outport
  wires:
  multiplier2/1 -> Binary Logic/2
  In2/1 -> multiplier2/1
  In4/1 -> Binary Logic1/2
  In1/1 -> Binary Logic/1
  multiplier4/1 -> Binary Logic1/1
  Binary Logic2/1 -> Port Out/1, Out1/1
  In3/1 -> multiplier4/1
  Port Out/1 -> Display5/1
  Binary Logic/1 -> Binary Logic2/1
  Binary Logic1/1 -> Binary Logic2/2

== system parallel/AES1 1/Round9/Subsystem8/Subsystem3/Mixcolumn2 ==
  In1 : Inport
  In2 : Inport  Port=2
  In3 : Inport  Port=3
  In4 : Inport  Port=4
  Binary Logic : shlslibv1/Math Functions/Binary Logic  syn_binlog_exp=a^b  synBlockType=primitive  synLatency=0  synBlockId=13
  Binary Logic1 : shlslibv1/Math Functions/Binary Logic  syn_binlog_exp=a^b  synBlockType=primitive  synLatency=0  synBlockId=13
  Binary Logic2 : shlslibv1/Math Functions/Binary Logic  syn_binlog_exp=a^b  synBlockType=primitive  synLatency=0  synBlockId=13
  Display5 : Display
      settings: Format=hex (Stored Integer)
  Port Out : shlslibv1/Ports & Subsystems/Port Out  syn_capture=on  syn_register=on  synBlockType=port  synLatency=1  synBlockId=1
  multiplier2 : shlslibv1/Memories/ROM  syn_rom_vec=multiplier2  syn_rom_auto_wl=on  syn_out_wl=8  syn_out_fl=0  syn_out_dt=unsigned  syn_out_sat=on  syn_out_rnd=on  syn_en_port=off  synBlockType=primitive  synLatency=1  synBlockId=62  syn_dual_port=off
  multiplier3 : shlslibv1/Memories/ROM  syn_rom_vec=multiplier3  syn_rom_auto_wl=on  syn_out_wl=8  syn_out_fl=0  syn_out_dt=unsigned  syn_out_sat=on  syn_out_rnd=on  syn_en_port=off  synBlockType=primitive  synLatency=1  synBlockId=62  syn_dual_port=off
  Out1 : Outport
  wires:
  In1/1 -> Binary Logic/1
  Binary Logic2/1 -> Port Out/1, Out1/1
  In4/1 -> multiplier3/1
  In3/1 -> multiplier2/1
  In2/1 -> Binary Logic/2
  multiplier2/1 -> Binary Logic1/1
  multiplier3/1 -> Binary Logic1/2
  Binary Logic/1 -> Binary Logic2/1
  Binary Logic1/1 -> Binary Logic2/2
  Port Out/1 -> Display5/1

== system parallel/AES1 1/Round9/Subsystem8/Subsystem3/Mixcolumn3 ==
  In1 : Inport
  In2 : Inport  Port=2
  In3 : Inport  Port=3
  In4 : Inport  Port=4
  Binary Logic : shlslibv1/Math Functions/Binary Logic  syn_binlog_exp=a^b  synBlockType=primitive  synLatency=0  synBlockId=13
  Binary Logic1 : shlslibv1/Math Functions/Binary Logic  syn_binlog_exp=a^b  synBlockType=primitive  synLatency=0  synBlockId=13
  Binary Logic2 : shlslibv1/Math Functions/Binary Logic  syn_binlog_exp=a^b  synBlockType=primitive  synLatency=0  synBlockId=13
  Display5 : Display
      settings: Format=hex (Stored Integer)
  Port Out : shlslibv1/Ports & Subsystems/Port Out  syn_capture=on  syn_register=on  synBlockType=port  synLatency=1  synBlockId=1
  multiplier1 : shlslibv1/Memories/ROM  syn_rom_vec=multiplier2  syn_rom_auto_wl=on  syn_out_wl=8  syn_out_fl=0  syn_out_dt=unsigned  syn_out_sat=on  syn_out_rnd=on  syn_en_port=off  synBlockType=primitive  synLatency=1  synBlockId=62  syn_dual_port=off
  multiplier4 : shlslibv1/Memories/ROM  syn_rom_vec=multiplier3  syn_rom_auto_wl=on  syn_out_wl=8  syn_out_fl=0  syn_out_dt=unsigned  syn_out_sat=on  syn_out_rnd=on  syn_en_port=off  synBlockType=primitive  synLatency=1  synBlockId=62  syn_dual_port=off
  Out1 : Outport
  wires:
  In2/1 -> Binary Logic/2
  multiplier1/1 -> Binary Logic1/2
  multiplier4/1 -> Binary Logic/1
  In3/1 -> Binary Logic1/1
  In1/1 -> multiplier4/1
  Binary Logic2/1 -> Port Out/1, Out1/1
  In4/1 -> multiplier1/1
  Port Out/1 -> Display5/1
  Binary Logic/1 -> Binary Logic2/1
  Binary Logic1/1 -> Binary Logic2/2
